simulink model "p2"  (R2024a)
settings: Solver=VariableStepAuto  StartTime=0.0  StopTime=10.0  RelTol=1e-3
undefined symbols (not defined in the file or in its folder): B
settings Model: Creator=majidsadeghinejad  LastModifiedBy=majidsadeghinejad

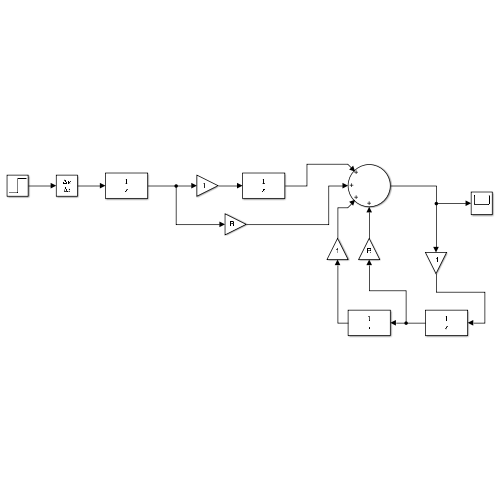
[thumbnail: Simulink's stored preview of the top-level diagram]
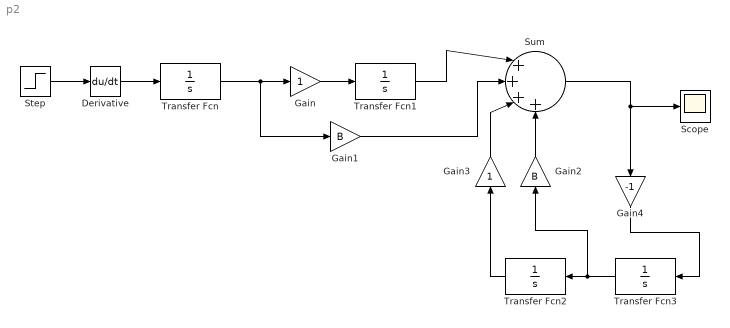
== system p2 ==
  Derivative : Derivative
  Gain : Gain
  Gain1 : Gain  Gain=B
  Gain2 : Gain  Gain=B
  Gain3 : Gain
  Gain4 : Gain  Gain=-1
  Scope : Scope
  Step : Step  Time=0.001  SampleTime=0
  Sum : Sum  Inputs=|++++
  Transfer Fcn{,1..3} (4 alike) : TransferFcn  Denominator=[1 0]
  wires:
  Transfer Fcn2/1 -> Gain3/1
  Sum/1 -> Gain4/1, Scope/1
  Transfer Fcn/1 -> Gain1/1, Gain/1
  Transfer Fcn3/1 -> Transfer Fcn2/1, Gain2/1
  Step/1 -> Derivative/1
  Gain2/1 -> Sum/4
  Derivative/1 -> Transfer Fcn/1
  Gain/1 -> Transfer Fcn1/1
  Gain4/1 -> Transfer Fcn3/1
  Gain3/1 -> Sum/3
  Gain1/1 -> Sum/2
  Transfer Fcn1/1 -> Sum/1
